simulink model "model_2"  (R2018b)
settings: Solver=VariableStepAuto  StartTime=0.0  StopTime=10.0  RelTol=1e-3
values from neighbouring files (symbols this model uses):
  A = total_intrest    (= 1.04)    [Capitalization.m]    (also in DiscretSystem.m = lamda(i); DiscreteVsContinues.m = expm(h*A))
  A_c = [0 1;-I -N]    [DiscreteVsContinues.m]
  B = 0    [Capitalization.m]    (also in DiscretSystem.m; DiscreteVsContinues.m = double(int(expm(z*A_c)*B_c,z,0,h)))
  B_c = [0;1]    [DiscreteVsContinues.m]
  C = 1    [Capitalization.m]    (also in DiscretSystem.m; DiscreteVsContinues.m = C_c)
  C_c = [1 0; 0 1]    [DiscreteVsContinues.m]
  D = 0    [Capitalization.m]    (also in DiscretSystem.m; DiscreteVsContinues.m = D_c)
  D_c = [0;0]    [DiscreteVsContinues.m]
  h = cap_rate    [Capitalization.m]    (also in DiscretSystem.m = 1; DiscreteVsContinues.m = 0.01)
  Start = 10000    [Capitalization.m]    (also in DiscretSystem.m = 10; DiscreteVsContinues.m = 5)
  Start_c = Start    (= 5)    [DiscreteVsContinues.m]
settings Model: Creator=bion  LastModifiedBy=bion

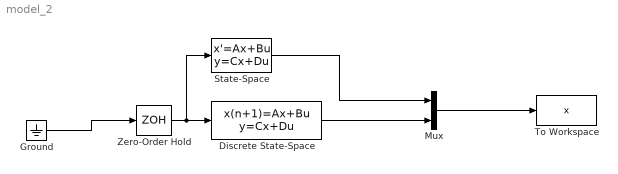
== system model_2 ==
  Discrete State-Space : DiscreteStateSpace  A=A  B=B  C=C  D=D  InitialCondition=Start  SampleTime=h
  Ground : Ground
  Mux : Mux  Inputs=2
  State-Space : StateSpace  A=A_c  B=B_c  C=C_c  D=D_c  InitialCondition=Start_c
  To Workspace : ToWorkspace  VariableName=x  SampleTime=-1
  Zero-Order Hold : ZeroOrderHold  SampleTime=h
  wires:
  Discrete State-Space/1 -> Mux/2
  Zero-Order Hold/1 -> State-Space/1, Discrete State-Space/1
  Ground/1 -> Zero-Order Hold/1
  State-Space/1 -> Mux/1
  Mux/1 -> To Workspace/1
